simulink model "mech_toroid"  (Simulink 6.0)
settings: Solver=ode45  StartTime=0.0  StopTime=150  RelTol=1e-3
PreLoadFcn:
  | mech_toroid_setup;
StartFcn:
  | mech_toroid_setup(gcs);
values from neighbouring files (symbols this model uses):
  m = 161    [mech_transmission_data.mat]
  N = 270    [mech_transmission_data.mat]
libraries: mblibv1 x9
settings Model: Creator=arnav  LastModifiedBy=batserve  ExtModeAutoUpdateStatusClock=off
settings DataIOCC: SignalLoggingName=logsOut  OutputOption=SpecifiedOutputTimes  OutputTimes=linspace(0,150,1000)
settings DebuggingCC: CheckExecutionContextPreStartOutputMsg=on  CheckExecutionContextRuntimeOutputMsg=on  SolverPrmCheckMsg=none
settings SimMechanicsCC: VisOnUpdateDiagram=on  VisDuringSimulation=on  VisConfigFile=mech_toroid_viz.mat

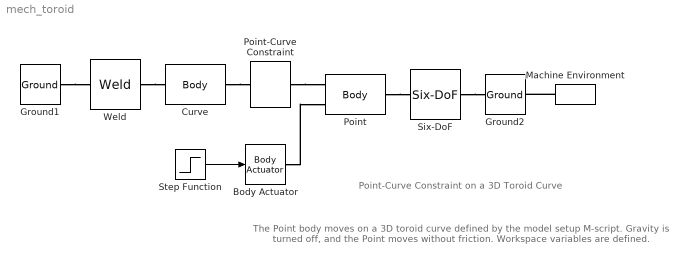
== system mech_toroid ==
  note: Point-Curve Constraint
      | on a 3D Toroid Curve
  note: The Point body moves on a 3D toroid curve defined
      | by the model setup M-script.  Gravity is turned off,
      | and the Point moves without friction.
      | Workspace variables are defined.
  Body Actuator : mblibv1/Sensors &  Actuators/Body Actuator  Opaque=on  PhysicalDomain=Mechanical  PortType=blob  ActuationStyle=Force  AngleUnits=deg  ArcVelocityUnits=deg/s  ArcAccelerationUnits=deg/s^2  CoordPositionUnits=m  VelocityUnits=m/s  AccelerationUnits=m/s^2  ForceUnits=N  TorqueUnits=N-m  ActiveIO=on  Width=3  DialogClass=MechanicalActuatorBlock  ReferenceFrame=Absolute (World)  Angle=off  CoordPosition=on  Force=on  Torque=off
  Curve : mblibv1/Bodies/Body  PhysicalDomain=mechanical  SubClassName=Unknown  LeftPortType=workingframe  RightPortType=workingframe  LConnTagsString=CS1  RConnTagsString=CS2  DialogClass=MechanicalBodyBlock  Mass=1  MassUnits=kg  InertiaUnits=kg*m^2  Inertia=eye(3)*5  Shape=Cylinder  ShapeDims=[1 1]  ShapeUnits=m  ShapeUse=false  Density=1  DensityUnits=kg/m^3  DensityUse=false  CG=Left$CG$[0 0 0]$CS1$CS1$m$[0 0 0]$Euler X-Y-Z$deg$WORLD$false  WorkingFrames=Left$CS1$[0 0 0]$WORLD$WORLD$m$[0 0 0]$Euler X-Y-Z$deg$WORLD$true#Right$CS2$[0 0 0]$CS1$CS1$m$[0 0 0]$Euler X-Y-Z$deg$WORLD$true
  Ground1 : mblibv1/Bodies/Ground  Opaque=on  LeftPortType=env  RightPortType=workingframe  PhysicalDomain=Mechanical  DialogClass=GroundBlock  CoordPosition=[0 0 0]  CoordPositionUnits=m  StateVectorMgrId=-1  MachineId=[0 0]  ShowEnvPort=off
  Ground2 : mblibv1/Bodies/Ground  Orientation=left  Opaque=on  LeftPortType=env  RightPortType=workingframe  PhysicalDomain=Mechanical  DialogClass=GroundBlock  CoordPosition=[0 0 0]  CoordPositionUnits=m  StateVectorMgrId=-1  MachineId=[0 0]  ShowEnvPort=on
  Machine Environment : mblibv1/Bodies/Machine Environment  Tag=Factory ground  Orientation=left  DialogController=MECH.DialogSource  Opaque=on  PortType=env  PhysicalDomain=Mechanical  DialogTemplateClass=MECH.MachineEnvironment  SyncWhenCopied=off  Gravity=[0 0 0]  GravityUnits=m/s^2  GravityAsSignal=off  Dimensionality=3D Only  AnalysisType=Forward dynamics  LinearAssemblyTolerance=1e-3  LinearAssemblyToleranceUnits=m  AngularAssemblyTolerance=1e-3  AngularAssemblyToleranceUnits=rad  ConstraintSolverType=Stabilizing  ConstraintRelTolerance=1e-4  ConstraintAbsTolerance=1e-4  UseRobustSingularityHandling=off  StatePerturbationType=Fixed  PerturbationSize=1e-5  VisualizeMachine=on
  Point : mblibv1/Bodies/Body  PhysicalDomain=mechanical  SubClassName=Unknown  LeftPortType=workingframe  RightPortType=workingframe  LConnTagsString=CS1|CG  RConnTagsString=CS2  DialogClass=MechanicalBodyBlock  Mass=1  MassUnits=kg  InertiaUnits=kg*m^2  Inertia=eye(3)  Shape=Cylinder  ShapeDims=[1 1]  ShapeUnits=m  ShapeUse=false  Density=1  DensityUnits=kg/m^3  DensityUse=false  CG=Left$CG$[0 0 0]$CS1$CS1$m$[0 0 0]$Euler X-Y-Z$deg$WORLD$true  WorkingFrames=Left$CS1$[toroid_X(1) toroid_Y(1) toroid_Z(1)]$WORLD$WORLD$m$[0 0 0]$Euler X-Y-Z$deg$WORLD$true#Right$CS2$[1 0 0]$CS1$CS1$m$[0 0 0]$Euler X-Y-Z$deg$WORLD$true
  Point-Curve Constraint : mblibv1/Constraints &  Drivers/Point-Curve Constraint  Orientation=left  PhysicalDomain=mechanical  SubClassName=Unknown  LeftPortType=blob  RightPortType=blob  LConnTagsString=__newl0  RConnTagsString=__newr0  DialogClass=PointCurveConstraint  Units=m  Xbreaks=toroid_X  Ybreaks=toroid_Y  Zbreaks=toroid_Z  EndConditions=periodic  CanExtrapolate=off  NumSAPorts=0
  Six-DoF : mblibv1/Joints/Six-DoF  PhysicalDomain=mechanical  SubClassName=Unknown  LeftPortType=blob  RightPortType=blob  LConnTagsString=__newl0  RConnTagsString=__newr0  NumSAPorts=0  CutJoint=off  MarkAsCut=off  Primitives=prismatic_prismatic_prismatic_spherical  PrimitiveProps=P1$WORLD$[1 0 0]$prismatic#P2$WORLD$[0 1 0]$prismatic#P3$WORLD$[0 0 1]$prismatic#S$WORLD$[0 0 0]$spherical  DialogClass=JointBlock
  Step Function : Step  Before=[-10 -10 -10]  After=0  SampleTime=0
  Weld : mblibv1/Joints/Weld  Orientation=left  PhysicalDomain=mechanical  SubClassName=Unknown  LeftPortType=blob  RightPortType=blob  LConnTagsString=__newl0  RConnTagsString=__newr0  NumSAPorts=0  CutJoint=off  MarkAsCut=off  Primitives=weld  PrimitiveProps=W$INERTIAL$[0 0 0]$weld  DialogClass=JointBlock
  wires:
  Step Function/1 -> Body Actuator/1
  connections:
  Machine Environment/RConn1 -- Ground2/LConn1
  Point/RConn1 -- Six-DoF/LConn1
  Six-DoF/RConn1 -- Ground2/RConn1
  Curve/RConn1 -- Point-Curve Constraint/RConn1
  Point-Curve Constraint/LConn1 -- Point/LConn1
  Ground1/RConn1 -- Weld/RConn1
  Weld/LConn1 -- Curve/LConn1
  Body Actuator/RConn1 -- Point/LConn2
